simulink library "mad_lib_template"  (R2019a)
settings: Solver=VariableStepAuto  StartTime=0.0  StopTime=10.0  RelTol=1e-3
values from neighbouring files (symbols this model uses):
  P_dt = 20e-3    (= 0.02)    [s6_data.m]
  P_p_c_2 = 83e-3    (= 0.083)    [p_mad_car.m]
  P_sim_dt = 2e-3    (= 0.002)    [s6_data.m]
undefined symbols (not defined in the file or in its folder): mbc_car_display, P_width
settings Model: Creator=ftraenkle  LastModifiedBy=ftraenkle

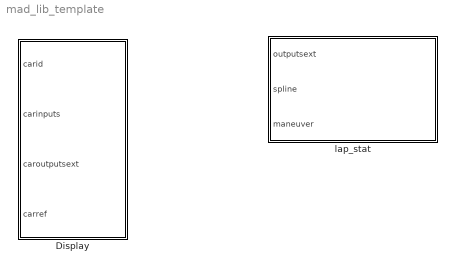
== system mad_lib_template ==
  Display : Subsystem
  lap_stat : Subsystem

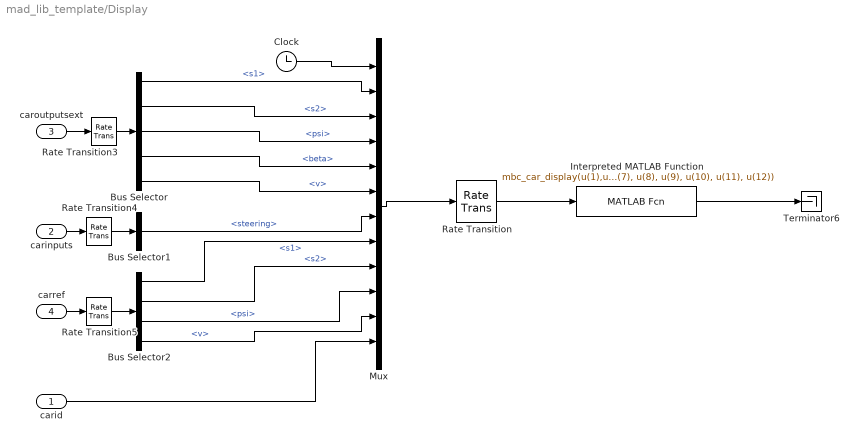
== system mad_lib_template/Display ==
  carid : Inport
  carinputs : Inport  Port=2
  caroutputsext : Inport  Port=3
  carref : Inport  Port=4
  Bus Selector : BusSelector  OutputSignals=s1,s2,psi,beta,v
  Bus Selector1 : BusSelector  OutputSignals=steering
  Bus Selector2 : BusSelector  OutputSignals=s1,s2,psi,v
  Clock : Clock
  Interpreted MATLAB Function : MATLABFcn  MATLABFcn=mbc_car_display(u(1),u(2),u(3),u(4),u(5), u(6), u(7), u(8), u(9), u(10), u(11), u(12))
  Mux : Mux  Inputs=12
  Rate Transition : RateTransition  OutPortSampleTime=P_display_dt
  Rate Transition3 : RateTransition
  Rate Transition4 : RateTransition
  Rate Transition5 : RateTransition
  Terminator6 : Terminator
  wires:
  Rate Transition5/1 -> Bus Selector2/1
  Rate Transition3/1 -> Bus Selector/1
  Rate Transition4/1 -> Bus Selector1/1
  carid/1 -> Mux/12
  Bus Selector2/1 -> Mux/8  "<s1>"
  Bus Selector2/2 -> Mux/9  "<s2>"
  Bus Selector2/3 -> Mux/10  "<psi>"
  Bus Selector2/4 -> Mux/11  "<v>"
  carref/1 -> Rate Transition5/1
  Bus Selector/5 -> Mux/6  "<v>"
  Bus Selector/4 -> Mux/5  "<beta>"
  Bus Selector1/1 -> Mux/7  "<steering>"
  carinputs/1 -> Rate Transition4/1
  Bus Selector/3 -> Mux/4  "<psi>"
  Bus Selector/2 -> Mux/3  "<s2>"
  Bus Selector/1 -> Mux/2  "<s1>"
  Clock/1 -> Mux/1
  Rate Transition/1 -> Interpreted MATLAB Function/1
  Mux/1 -> Rate Transition/1
  Interpreted MATLAB Function/1 -> Terminator6/1
  caroutputsext/1 -> Rate Transition3/1

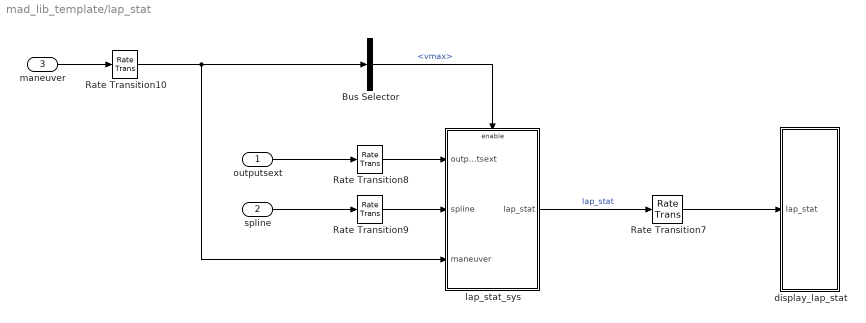
== system mad_lib_template/lap_stat ==
  outputsext : Inport
  spline : Inport  Port=2
  maneuver : Inport  Port=3
  Bus Selector : BusSelector  OutputSignals=vmax
  Rate Transition10 : RateTransition
  Rate Transition7 : RateTransition  OutPortSampleTime=P_display_dt
  Rate Transition8 : RateTransition
  Rate Transition9 : RateTransition
  display_lap_stat : Subsystem
  lap_stat_sys : Subsystem
  wires:
  Rate Transition10/1 -> Bus Selector/1, lap_stat_sys/3(maneuver)
  Rate Transition9/1 -> lap_stat_sys/2(spline)
  Rate Transition8/1 -> lap_stat_sys/1(outputsext)
  Rate Transition7/1 -> display_lap_stat/1(lap_stat)
  lap_stat_sys/1(lap_stat) -> Rate Transition7/1  "lap_stat"
  spline/1 -> Rate Transition9/1
  maneuver/1 -> Rate Transition10/1
  outputsext/1 -> Rate Transition8/1
  Bus Selector/1 -> lap_stat_sys/Enable  "<vmax>"

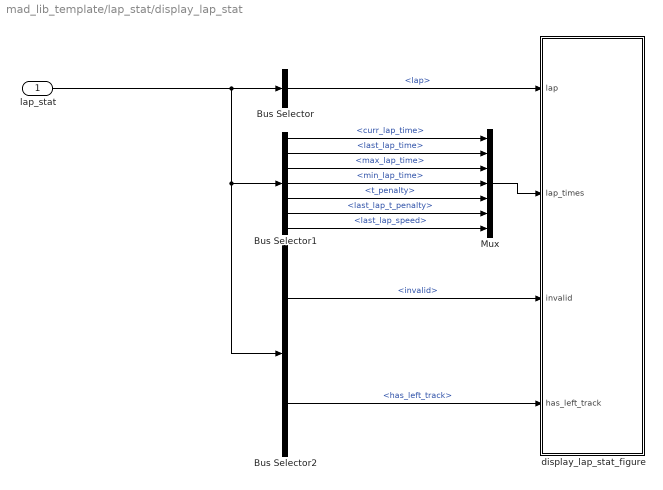
== system mad_lib_template/lap_stat/display_lap_stat ==
  lap_stat : Inport
  Bus Selector : BusSelector  OutputSignals=lap
  Bus Selector1 : BusSelector  OutputSignals=curr_lap_time,last_lap_time,max_lap_time,min_lap_time,t_penalty,last_lap_t_penalty,last_lap_speed
  Bus Selector2 : BusSelector  OutputSignals=invalid,has_left_track
  Mux : Mux  Inputs=7
  display_lap_stat_figure : MATLAB Function  TreatAsAtomicUnit=on
  wires:
  Bus Selector1/7 -> Mux/7  "<last_lap_speed>"
  Bus Selector1/6 -> Mux/6  "<last_lap_t_penalty>"
  Bus Selector1/5 -> Mux/5  "<t_penalty>"
  lap_stat/1 -> Bus Selector/1, Bus Selector1/1, Bus Selector2/1
  Bus Selector2/2 -> display_lap_stat_figure/4(has_left_track)  "<has_left_track>"
  Bus Selector2/1 -> display_lap_stat_figure/3(invalid)  "<invalid>"
  Bus Selector1/4 -> Mux/4  "<min_lap_time>"
  Bus Selector/1 -> display_lap_stat_figure/1(lap)  "<lap>"
  Mux/1 -> display_lap_stat_figure/2(lap_times)
  Bus Selector1/3 -> Mux/3  "<max_lap_time>"
  Bus Selector1/1 -> Mux/1  "<curr_lap_time>"
  Bus Selector1/2 -> Mux/2  "<last_lap_time>"

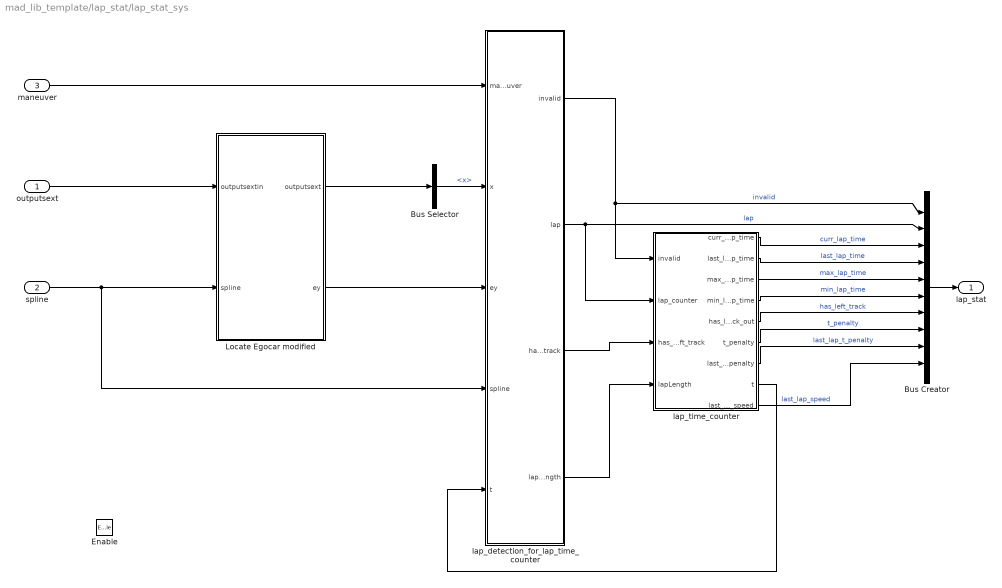
== system mad_lib_template/lap_stat/lap_stat_sys ==
  outputsext : Inport
  spline : Inport  Port=2
  maneuver : Inport  Port=3
  Enable : EnablePort  StatesWhenEnabling=reset
  Bus Creator : BusCreator  Inputs=10
  Bus Selector : BusSelector  OutputSignals=x
  Locate Egocar modified : Subsystem  SystemSampleTime=P_sim_dt
  lap_detection_for_lap_time_counter : Subsystem  SystemSampleTime=P_sim_dt
  lap_time_counter : Subsystem  SystemSampleTime=P_sim_dt
  lap_stat : Outport
  wires:
  lap_detection_for_lap_time_counter/4(lapLength) -> lap_time_counter/4(lapLength)
  lap_time_counter/9(last_lap_speed) -> Bus Creator/10  "last_lap_speed"
  lap_time_counter/7(last_lap_t_penalty) -> Bus Creator/9  "last_lap_t_penalty"
  lap_time_counter/6(t_penalty) -> Bus Creator/8  "t_penalty"
  lap_time_counter/5(has_left_track_out) -> Bus Creator/7  "has_left_track"
  lap_detection_for_lap_time_counter/1(invalid) -> Bus Creator/1, lap_time_counter/1(invalid)  "invalid"
  lap_detection_for_lap_time_counter/3(has_left_track) -> lap_time_counter/3(has_left_track)
  Locate Egocar modified/2(ey) -> lap_detection_for_lap_time_counter/3(ey)
  Bus Creator/1 -> lap_stat/1
  lap_time_counter/3(max_lap_time) -> Bus Creator/5  "max_lap_time"
  lap_time_counter/4(min_lap_time) -> Bus Creator/6  "min_lap_time"
  lap_time_counter/1(curr_lap_time) -> Bus Creator/3  "curr_lap_time"
  lap_time_counter/2(last_lap_time) -> Bus Creator/4  "last_lap_time"
  lap_time_counter/8(t) -> lap_detection_for_lap_time_counter/5(t)
  Locate Egocar modified/1(outputsext) -> Bus Selector/1
  Bus Selector/1 -> lap_detection_for_lap_time_counter/2(x)  "<x>"
  spline/1 -> Locate Egocar modified/2(spline), lap_detection_for_lap_time_counter/4(spline)
  outputsext/1 -> Locate Egocar modified/1(outputsextin)
  maneuver/1 -> lap_detection_for_lap_time_counter/1(maneuver)
  lap_detection_for_lap_time_counter/2(lap) -> Bus Creator/2, lap_time_counter/2(lap_counter)  "lap"

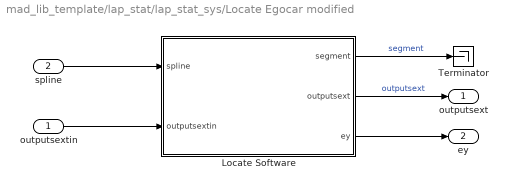
== system mad_lib_template/lap_stat/lap_stat_sys/Locate Egocar modified ==
  outputsextin : Inport
  spline : Inport  Port=2
  Locate Software : Subsystem  SystemSampleTime=P_dt
  Terminator : Terminator
  outputsext : Outport
  ey : Outport  Port=2
  wires:
  Locate Software/3(ey) -> ey/1
  spline/1 -> Locate Software/1(spline)
  outputsextin/1 -> Locate Software/2(outputsextin)
  Locate Software/2(outputsext) -> outputsext/1  "outputsext"
  Locate Software/1(segment) -> Terminator/1  "segment"

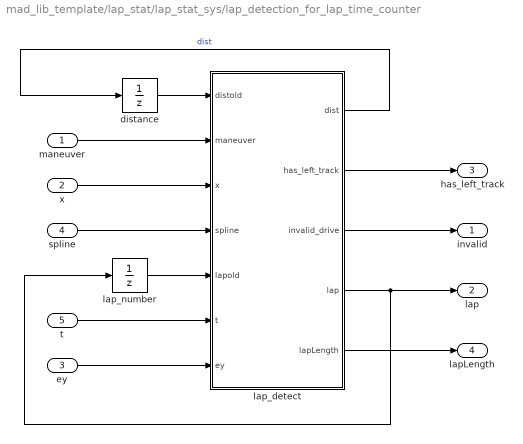
== system mad_lib_template/lap_stat/lap_stat_sys/lap_detection_for_lap_time_counter ==
  maneuver : Inport
  x : Inport  Port=2
  ey : Inport  Port=3
  spline : Inport  Port=4
  t : Inport  Port=5
  distance : UnitDelay  InitialCondition=-inf  SampleTime=-1  HasFrameUpgradeWarning=on
  lap_detect : MATLAB Function  TreatAsAtomicUnit=on
  lap_number : UnitDelay  InitialCondition=uint32(0)  SampleTime=-1  HasFrameUpgradeWarning=on
  invalid : Outport
  lap : Outport  Port=2
  has_left_track : Outport  Port=3
  lapLength : Outport  Port=4
  wires:
  lap_detect/5(lapLength) -> lapLength/1
  lap_detect/3(invalid_drive) -> invalid/1
  lap_detect/2(has_left_track) -> has_left_track/1
  ey/1 -> lap_detect/7(ey)
  t/1 -> lap_detect/6(t)
  distance/1 -> lap_detect/1(distold)
  lap_number/1 -> lap_detect/5(lapold)
  lap_detect/4(lap) -> lap/1, lap_number/1
  x/1 -> lap_detect/3(x)
  spline/1 -> lap_detect/4(spline)
  lap_detect/1(dist) -> distance/1  "dist"
  maneuver/1 -> lap_detect/2(maneuver)

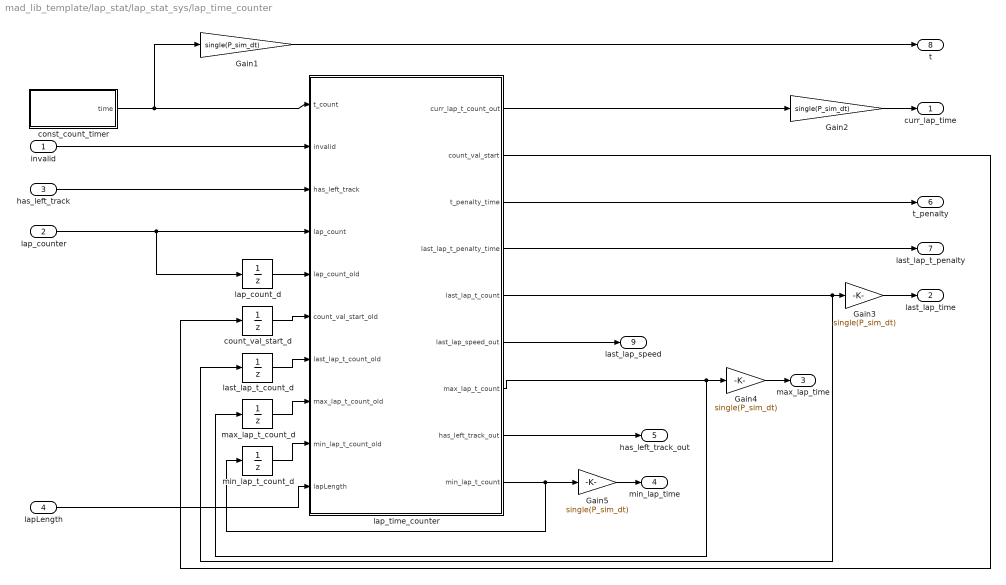
== system mad_lib_template/lap_stat/lap_stat_sys/lap_time_counter ==
  invalid : Inport
  lap_counter : Inport  Port=2
  has_left_track : Inport  Port=3
  lapLength : Inport  Port=4
  Gain{1..5} (5 alike) : Gain  Gain=single(P_sim_dt)  OutDataTypeStr=single
  const_count_timer : Subsystem
  count_val_start_d : UnitDelay  InitialCondition=uint32(0)  SampleTime=-1  HasFrameUpgradeWarning=on
  lap_count_d : UnitDelay  InitialCondition=uint32(0)  SampleTime=-1  HasFrameUpgradeWarning=on
  lap_time_counter : MATLAB Function  TreatAsAtomicUnit=on
  last_lap_t_count_d : UnitDelay  InitialCondition=uint32(intmax('uint32'))  SampleTime=-1  HasFrameUpgradeWarning=on
  max_lap_t_count_d : UnitDelay  InitialCondition=uint32(0)  SampleTime=-1  HasFrameUpgradeWarning=on
  min_lap_t_count_d : UnitDelay  InitialCondition=uint32(intmax('uint32'))  SampleTime=-1  HasFrameUpgradeWarning=on
  curr_lap_time : Outport
  last_lap_time : Outport  Port=2
  max_lap_time : Outport  Port=3
  min_lap_time : Outport  Port=4
  has_left_track_out : Outport  Port=5
  t_penalty : Outport  Port=6
  last_lap_t_penalty : Outport  Port=7
  t : Outport  Port=8
  last_lap_speed : Outport  Port=9
  wires:
  lapLength/1 -> lap_time_counter/10(lapLength)
  lap_time_counter/6(last_lap_speed_out) -> last_lap_speed/1
  invalid/1 -> lap_time_counter/2(invalid)
  lap_time_counter/4(last_lap_t_penalty_time) -> last_lap_t_penalty/1
  lap_time_counter/3(t_penalty_time) -> t_penalty/1
  lap_time_counter/8(has_left_track_out) -> has_left_track_out/1
  has_left_track/1 -> lap_time_counter/3(has_left_track)
  lap_time_counter/9(min_lap_t_count) -> Gain5/1, min_lap_t_count_d/1
  Gain5/1 -> min_lap_time/1
  Gain4/1 -> max_lap_time/1
  lap_time_counter/7(max_lap_t_count) -> max_lap_t_count_d/1, Gain4/1
  min_lap_t_count_d/1 -> lap_time_counter/9(min_lap_t_count_old)
  max_lap_t_count_d/1 -> lap_time_counter/8(max_lap_t_count_old)
  Gain3/1 -> last_lap_time/1
  Gain2/1 -> curr_lap_time/1
  Gain1/1 -> t/1
  lap_time_counter/5(last_lap_t_count) -> Gain3/1, last_lap_t_count_d/1
  last_lap_t_count_d/1 -> lap_time_counter/7(last_lap_t_count_old)
  lap_time_counter/1(curr_lap_t_count_out) -> Gain2/1
  lap_count_d/1 -> lap_time_counter/5(lap_count_old)
  count_val_start_d/1 -> lap_time_counter/6(count_val_start_old)
  lap_counter/1 -> lap_time_counter/4(lap_count), lap_count_d/1
  lap_time_counter/2(count_val_start) -> count_val_start_d/1
  const_count_timer/1(time) -> lap_time_counter/1(t_count), Gain1/1

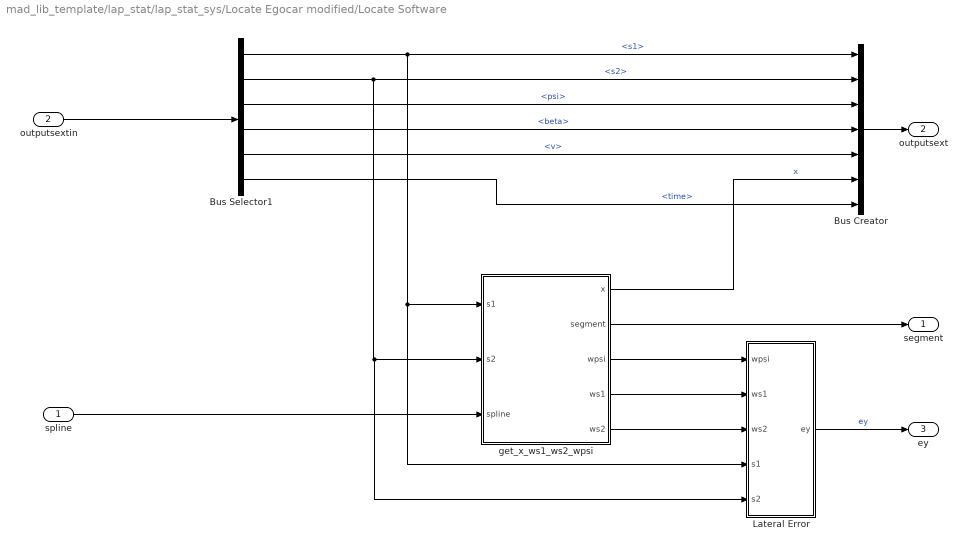
== system mad_lib_template/lap_stat/lap_stat_sys/Locate Egocar modified/Locate Software ==
  spline : Inport
  outputsextin : Inport  Port=2
  Bus Creator : BusCreator  Inputs=7  OutDataTypeStr=Bus: CAROUTPUTSEXT  NonVirtualBus=on
  Bus Selector1 : BusSelector  OutputSignals=s1,s2,psi,beta,v,time
  Lateral Error : Subsystem
  get_x_ws1_ws2_wpsi : MATLAB Function  TreatAsAtomicUnit=on
  segment : Outport
  outputsext : Outport  Port=2
  ey : Outport  Port=3
  wires:
  Lateral Error/1(ey) -> ey/1  "ey"
  get_x_ws1_ws2_wpsi/5(ws2) -> Lateral Error/3(ws2)
  get_x_ws1_ws2_wpsi/4(ws1) -> Lateral Error/2(ws1)
  get_x_ws1_ws2_wpsi/3(wpsi) -> Lateral Error/1(wpsi)
  Bus Selector1/6 -> Bus Creator/7  "<time>"
  outputsextin/1 -> Bus Selector1/1
  Bus Selector1/2 -> get_x_ws1_ws2_wpsi/2(s2), Lateral Error/5(s2), Bus Creator/2  "<s2>"
  Bus Selector1/4 -> Bus Creator/4  "<beta>"
  Bus Selector1/5 -> Bus Creator/5  "<v>"
  Bus Creator/1 -> outputsext/1
  Bus Selector1/3 -> Bus Creator/3  "<psi>"
  get_x_ws1_ws2_wpsi/1(x) -> Bus Creator/6  "x"
  Bus Selector1/1 -> Lateral Error/4(s1), get_x_ws1_ws2_wpsi/1(s1), Bus Creator/1  "<s1>"
  spline/1 -> get_x_ws1_ws2_wpsi/3(spline)
  get_x_ws1_ws2_wpsi/2(segment) -> segment/1

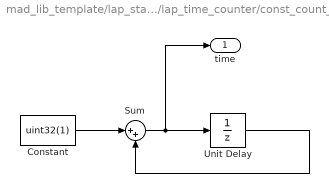
== system mad_lib_template/lap_stat/lap_stat_sys/lap_time_counter/const_count_timer ==
  Constant : Constant  Value=uint32(1)  SampleTime=-1
  Sum : Sum  Inputs=|++
  Unit Delay : UnitDelay  InitialCondition=uint32(0)  SampleTime=-1  HasFrameUpgradeWarning=on
  time : Outport
  wires:
  Unit Delay/1 -> Sum/2
  Constant/1 -> Sum/1
  Sum/1 -> Unit Delay/1, time/1

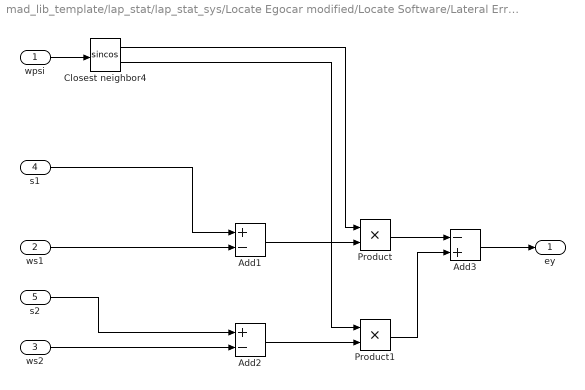
== system mad_lib_template/lap_stat/lap_stat_sys/Locate Egocar modified/Locate Software/Lateral Error ==
  wpsi : Inport
  ws1 : Inport  Port=2
  ws2 : Inport  Port=3
  s1 : Inport  Port=4
  s2 : Inport  Port=5
  Add1 : Sum  Inputs=+-
  Add2 : Sum  Inputs=+-
  Add3 : Sum  Inputs=-+
  Closest neighbor4 : Trigonometry  Operator=sincos
  Product : Product
  Product1 : Product
  ey : Outport
  wires:
  Product/1 -> Add3/1
  ws2/1 -> Add2/2
  s1/1 -> Add1/1
  Closest neighbor4/2 -> Product1/1
  s2/1 -> Add2/1
  Add1/1 -> Product/2
  Product1/1 -> Add3/2
  wpsi/1 -> Closest neighbor4/1
  Add3/1 -> ey/1
  Closest neighbor4/1 -> Product/1
  ws1/1 -> Add1/2
  Add2/1 -> Product1/2

== matlab function mad_lib_template/lap_stat/display_lap_stat/display_lap_stat_figure ==
  data: lap input; lap_times input; invalid input; has_left_track input
function disp_lap_stat(lap, lap_times, invalid, has_left_track)

%coder.extrinsic('text');
%coder.extrinsic('sprintf');

% Static
persistent t_hand fig_track_hand fig_statinfo_hand;

% At first step init
if isempty(t_hand)
    % Get figure handle of track
    fig_track_hand    = gcf;    
    
    % Open figure (save handle) of status window 
    fig_statinfo_hand = figure(2);
    
    % Use normalized metric and set size and position of info window
    set(fig_statinfo_hand, 'Units', 'Normalized', 'Position', [0, 0.4, 0.44, 0.2]);
    
    % Clear the figure and modify axis properties
    clf;
    axis([ 0 1 0 1 ]);
    axis manual;
    axis off;
    
    % Set initial text
    t_hand = text(0., 0.5, '', 'FontName', 'FixedWidth', 'FontSize', 12);
end

%set(0, 'CurrentFigure', fig_statinfo_hand);

% str1 & str2 are stus strings, reset them
str1=''; str2='';

% Check status and set strings
if has_left_track
    str1 = 'off-track';
end

if invalid 
    str2 = 'fatal-crash'; 
end

% Set Info text
set(t_hand, 'String', {['Lap #' ,sprintf('%u', lap+1)], ...
                       ['Current lap time     : ', sprintf('%5.3fs', lap_times(1))], ... 
                       ['Current penalty time : ', sprintf('%5.3fs', lap_times(5))], ... 
                       ['Last lap time        : ', sprintf('%5.3fs', lap_times(2))], ...
                       ['Last penalty time    : ', sprintf('%5.3fs', lap_times(6))], ...
                       ['Last lap avg. speed  : ', sprintf('%5.3fm/s', lap_times(7))], ...
                       ['Last lap+penalty time: ', sprintf('%5.3fs', lap_times(2)+lap_times(6))], ...
                       ['Max lap+penalty time : ', sprintf('%5.3fs', lap_times(3))], ...
                       ['Min lap+penalty time : ', sprintf('%5.3fs', lap_times(4))], ...
                       ['Status               : ', sprintf('%s , %s', str2, str1)], ...
                       });

% Track window -> current window (it has lost focus above)
set(0, 'CurrentFigure', fig_track_hand);

end

== matlab function mad_lib_template/lap_stat/lap_stat_sys/lap_time_counter/lap_time_counter ==
  data: t_count input uint32; invalid input uint8; has_left_track input uint8; curr_lap_t_count_out output size=1; count_val_start output uint32; t_penalty_time output; last_lap_t_penalty_time output; last_lap_t_count output uint32 size=1; last_lap_speed_out output; lap_count input; lap_count_old input; count_val_start_old input uint32; last_lap_t_count_old input uint32; max_lap_t_count_old input uint32; min_lap_t_count_old input uint32; lapLength input; max_lap_t_count output uint32 size=1; has_left_track_out output; min_lap_t_count output uint32 size=1; P_sim_dt parameter
function [curr_lap_t_count_out, count_val_start, t_penalty_time, last_lap_t_penalty_time, last_lap_t_count, last_lap_speed_out, max_lap_t_count, has_left_track_out, min_lap_t_count]= lap_time_counter(t_count, invalid, has_left_track, lap_count, lap_count_old, count_val_start_old, last_lap_t_count_old, max_lap_t_count_old, min_lap_t_count_old, lapLength, P_sim_dt)

P_penalty_time_coeff = single(1);

% Static
persistent leave_track_t_counter last_lap_penalty_t_count curr_lap_t_count last_lap_speed;


% At first: step init static
if isempty(leave_track_t_counter)
    leave_track_t_counter           = uint32(0);
    last_lap_penalty_t_count        = uint32(0);
    curr_lap_t_count                = uint32(0);
    last_lap_speed = single(0);
end


% Not modified up to now
has_left_track_out                  = has_left_track;

 % Init output beeing within a lap
count_val_start                     = count_val_start_old;
last_lap_t_count                    = last_lap_t_count_old;
max_lap_t_count                     = max_lap_t_count_old;
min_lap_t_count                     = min_lap_t_count_old;

% If no fatal crash
if ~invalid
    
    % Current lap time count
    curr_lap_t_count                = t_count - count_val_start_old;   % time of current lap
    

    % If car has left the track (sum of leaving track time per lap)
    if has_left_track
        leave_track_t_counter       = leave_track_t_counter + uint32(1);
    end

    % New lap starts or first step
    if lap_count ~= lap_count_old ||  ~count_val_start_old  

        % Not at first lap
        if count_val_start_old ~= 0

            % Save last lap time and add penalty time
            last_lap_penalty_t_count= uint32(double(leave_track_t_counter)*P_penalty_time_coeff); 
            last_lap_t_count        = curr_lap_t_count;
            total_lap_t_count = last_lap_t_count + last_lap_penalty_t_count;            
            if total_lap_t_count > max_lap_t_count
                max_lap_t_count     = total_lap_t_count;
            end

            if total_lap_t_count < min_lap_t_count
                min_lap_t_count     = total_lap_t_count;
            end
            last_lap_speed = single(lapLength) / (single(last_lap_t_count) * single(P_sim_dt));
        end

        % Restart counting
        count_val_start             = t_count;      % Save counter value at the beginning of the lap
        leave_track_t_counter       = uint32(0);    % Reset leave track counter because o startin new lap
    end

end

% Penalty time to display
t_penalty_time                      = single(leave_track_t_counter)*P_penalty_time_coeff*P_sim_dt;

% Last lap penalty time to display 
last_lap_t_penalty_time             = single(last_lap_penalty_t_count)*P_sim_dt;

% Last lap time count (Note: curr_lap_t_count is static)
curr_lap_t_count_out                = curr_lap_t_count;

% Last lap speed (Note: last_lap_speed is static)
last_lap_speed_out = last_lap_speed;

end

== matlab function mad_lib_template/lap_stat/lap_stat_sys/lap_detection_for_lap_time_counter/lap_detect ==
  data: distold input; dist output; has_left_track output size=1; invalid_drive output size=1; maneuver input; x input; spline input; lap output size=1; lapold input uint32; t input; ey input; P_width parameter; P_p_c_2 parameter; lapLength output
function [ dist, has_left_track, invalid_drive, lap, lapLength ] = lap_detect(distold, maneuver, x, spline, lapold, t, ey, P_width, P_p_c_2)

% Static
persistent x0 invalid;

% Init variables
P_ey_leave          = (P_width-P_p_c_2) * 0.5;
P_ey_leave_max      = (P_width+P_p_c_2) * 0.5;
P_tstart_lap_detec  = 0.2;
lap                 = uint32(0);
has_left_track      = uint8(1);


% At first step
if isempty(x0)
    % Save initial value
    x0 = x;
    
    % Valid driving test
    invalid         = uint8(0);  
end

% Lap length
lapLength =  maneuver.xManeuverEnd; 

% circular track: get track len
if spline.periodic && spline.breakslen > 0   
    lapLength = spline.points(1, spline.breakslen);
end 

dist = lapLength - (x-x0);

% Has left the track?
if abs(ey) <= P_ey_leave
    has_left_track = uint8(0);
end

% Has left the track too far? Invalid driving test?
if abs(ey) > P_ey_leave_max
    invalid = uint8(1);
end

invalid_drive = invalid;

% Calc control deviation and lap count
if spline.periodic && spline.breakslen > 0
    % circular track
    
    %lapLength = spline.points(1, spline.breakslen);
    
    % adjust control deviation
    if dist < -0.5 * lapLength
        dist = dist + lapLength;
    elseif dist > 0.5 * lapLength
        dist = dist - lapLength;
    end
    
    % Skip lap detection for P_tstart_lap_detec sec
    if t > P_tstart_lap_detec 
        
        lap = lapold;
        if maneuver.vmax > 0
            % forward driving
            if distold >= 0 && distold < lapLength * 0.25 && dist < 0
                lap = lap + uint32(1);
            end
        elseif maneuver.vmax < 0
            % reverse driving
            if distold <= 0 && distold > lapLength * 0.25 && dist > 0
                lap = lap + uint32(1);
            end
        end    
    end
end
if maneuver.vmax < 0
    dist = -dist; % one case for forward and reverse driving
end
end

== matlab function mad_lib_template/lap_stat/lap_stat_sys/Locate Egocar modified/Locate Software/get_x_ws1_ws2_wpsi ==
  data: s1 input; x output; s2 input; spline input; segment output int32; wpsi output; ws1 output; ws2 output
function [ x, segment, wpsi, ws1, ws2] = get_x_ws1_ws2_wpsi(s1, s2, spline)
%#codegen
[ w, widx ] = mbc_spline_get_reference([ s1; s2 ], spline.breakslen, spline.points, spline.coefs, spline.periodic, 0, 0);
x = w(1);
if widx > 0
    segment = int32(spline.segments(widx));
else
    segment = int32(-1);
end

ws1 = w(3);
ws2 = w(4); 
wpsi = w(2);

end
